simulink model "pendulum_model1"  (Simulink 7.4)
settings: Solver=ode45  StartTime=0.0  StopTime=10.0  MaxStep=0.01  RelTol=1e-3
undefined symbols (not defined in the file): g, L, theta0
settings Model: Creator=m136852  LastModifiedBy=m136852
settings DataIOCC: LimitDataPoints=off  TimeSaveName=t

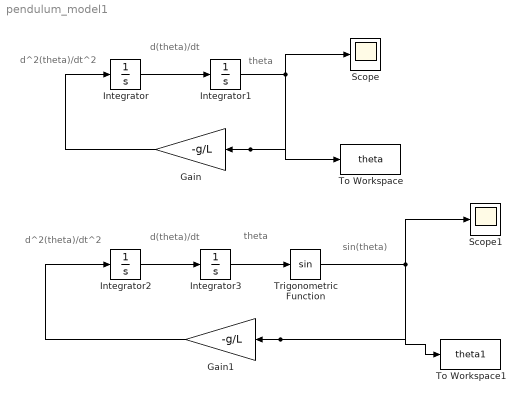
== system pendulum_model1 ==
  note: d^2(theta)/dt^2
  note: d(theta)/dt
  note: theta
  note: d^2(theta)/dt^2
  note: d(theta)/dt
  note: theta
  note: sin(theta)
  Gain : Gain  Gain=-g/L  ParameterDataType=fixdt(1, 16)  ParameterScaling=2^0  OutDataType=fixdt(1, 16)  OutScaling=2^0
  Gain1 : Gain  Gain=-g/L  ParameterDataType=fixdt(1, 16)  ParameterScaling=2^0  OutDataType=fixdt(1, 16)  OutScaling=2^0
  Integrator : Integrator
  Integrator1 : Integrator  InitialCondition=theta0*(pi/180)
  Integrator2 : Integrator
  Integrator3 : Integrator  InitialCondition=theta0*(pi/180)
  Scope : Scope
  Scope1 : Scope
  To Workspace : ToWorkspace  VariableName=theta  SampleTime=-1  SaveFormat=Array
  To Workspace1 : ToWorkspace  VariableName=theta1  SampleTime=-1  SaveFormat=Array
  Trigonometric Function : Trigonometry
  wires:
  Integrator1/1 -> Gain/1, To Workspace/1, Scope/1
  Integrator/1 -> Integrator1/1
  Gain/1 -> Integrator/1
  Integrator3/1 -> Trigonometric Function/1
  Integrator2/1 -> Integrator3/1
  Gain1/1 -> Integrator2/1
  Trigonometric Function/1 -> Gain1/1, To Workspace1/1, Scope1/1
